simulink model "developsim"  (R2013b)
settings: Solver=ode45  StartTime=0.0  StopTime=20  RelTol=1e-3
values from neighbouring files (symbols this model uses):
  b = 0.1    [QRrunfile.m]    (also in develop.m)
  d = 0.1    [QRrunfile.m]    (also in develop.m)
  dphi0 = 0    [develop.m]
  dpsi0 = 0    [develop.m]
  dtheta0 = 0    [develop.m]
  dx0 = 0    [QRrunfile.m]    (also in develop.m)
  dy0 = 0    [QRrunfile.m]    (also in develop.m)
  dz0 = 0    [QRrunfile.m]    (also in develop.m)
  e3 = [0;0;1]    [QRrunfile.m]
  g = 9.81    [QRrunfile.m]    (also in develop.m)
  I = diag([Ixx Iyy Izz])    [QRrunfile.m]    (also in develop.m)
  Ir = 0.5    [QRrunfile.m]    (also in develop.m)
  Ixx = 0.0820    (= 0.082)    [QRrunfile.m]    (also in develop.m = 1.5)
  Iyy = 0.0845    [QRrunfile.m]    (also in develop.m = 1.5)
  Izz = .1377    (= 0.1377)    [QRrunfile.m]    (also in develop.m = 1.5)
  kOmega = kOmega_phi*eye(3)    [QRrunfile.m]
  kR = kR_phi*eye(3)    [QRrunfile.m]
  l = 0.315    [QRrunfile.m]    (also in develop.m = 0.12)
  m = 4.34    [QRrunfile.m]    (also in develop.m = 0.42)
  phi0 = 0    [develop.m]
  psi0 = 0    [develop.m]
  theta0 = 0    [develop.m]
  x0 = 0    [QRrunfile.m]    (also in develop.m)
  y0 = 0    [QRrunfile.m]    (also in develop.m)
  z0 = 0    [QRrunfile.m]    (also in develop.m)
libraries: dspsrcs4 x9, simulink x1
settings Model: Creator=Nam  LastModifiedBy=Nam
settings DebuggingCC: SolverPrmCheckMsg=none

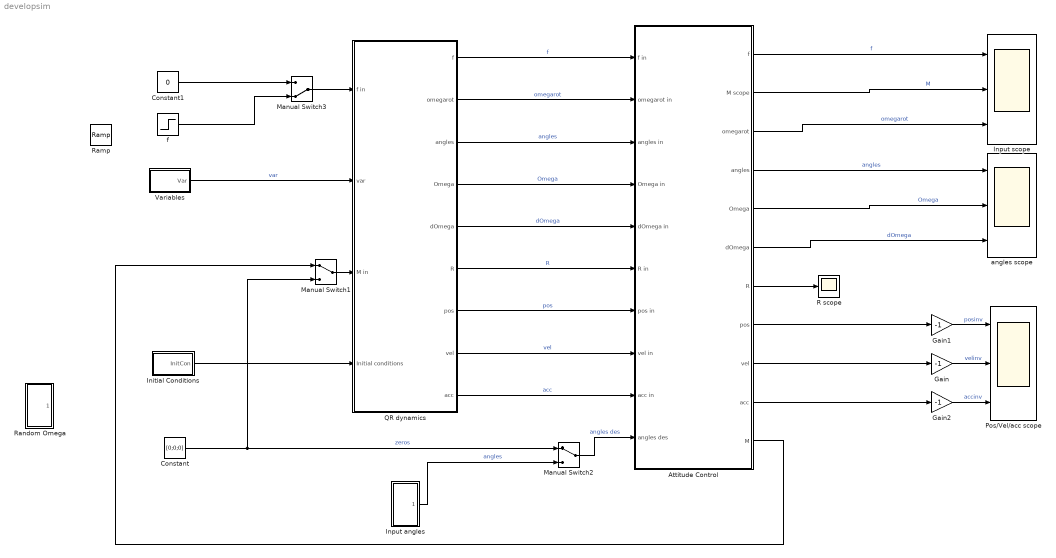
== system developsim ==
  Attitude Control : Subsystem
  Constant : Constant  Value=[0;0;0]
  Constant1 : Constant  Value=0
  Gain : Gain  Gain=-1
  Gain1 : Gain  Gain=-1
  Gain2 : Gain  Gain=-1
  Initial Conditions : Subsystem
      mask Display: disp('Initial\nConditions')
  Input angles : Subsystem
  Input scope : Scope  NumInputPorts=3
      settings: ShowLegends=on  YMin=3.91419~-1.75e+07~0  YMax=4.32621~2.5e+06~27500  SaveName=Scopeinputs
  Manual Switch1 : ManualSwitch
  Manual Switch2 : ManualSwitch
  Manual Switch3 : ManualSwitch  CurrentSetting=0
  Pos/Vel/acc scope : Scope  NumInputPorts=3
      settings: ShowLegends=on  YMin=-5~-5~-5  YMax=5~5~5  SaveName=Scopepos  SampleInput=on
  QR dynamics : Subsystem
  R scope : Scope
      settings: ShowLegends=on
  Ramp : simulink/Sources/Ramp  slope=.05  start=0  X0=m*g
  Random Omega : Subsystem
  Variables : Subsystem
      mask Display: disp('Variables')
  angles scope : Scope  NumInputPorts=3
      settings: ShowLegends=on  YMin=-5~-5~-5  YMax=5~5~5  SaveName=Scopeangles
  f : Step  Time=0  After=m*g  SampleTime=0
  wires:
  f/1 -> Manual Switch3/2
  Variables/1(Var) -> QR dynamics/2(var)  "var"
  Constant/1 -> Manual Switch2/1, Manual Switch1/2  "zeros"
  Initial Conditions/1(InitCon) -> QR dynamics/4(Initial conditions)
  QR dynamics/1(f) -> Attitude Control/1(f in)  "f"
  QR dynamics/2(omegarot) -> Attitude Control/2(omegarot in)  "omegarot"
  QR dynamics/3(angles) -> Attitude Control/3(angles in)  "angles"
  QR dynamics/5(dOmega) -> Attitude Control/5(dOmega in)  "dOmega"
  QR dynamics/6(R) -> Attitude Control/6(R in)  "R"
  QR dynamics/7(pos) -> Attitude Control/7(pos in)  "pos"
  QR dynamics/8(vel) -> Attitude Control/8(vel in)  "vel"
  QR dynamics/9(acc) -> Attitude Control/9(acc in)  "acc"
  Attitude Control/2(M scope) -> Input scope/2  "M"
  Attitude Control/3(omegarot) -> Input scope/3  "omegarot"
  Attitude Control/9(vel) -> Gain/1
  Attitude Control/7(R) -> R scope/1
  Attitude Control/10(acc) -> Gain2/1
  Attitude Control/8(pos) -> Gain1/1
  Attitude Control/1(f) -> Input scope/1  "f"
  Gain1/1 -> Pos/Vel/acc scope/1  "posinv"
  Gain/1 -> Pos/Vel/acc scope/2  "velinv"
  Gain2/1 -> Pos/Vel/acc scope/3  "accinv"
  Manual Switch1/1 -> QR dynamics/3(M in)
  Input angles/1(Out1) -> Manual Switch2/2  "angles"
  Manual Switch2/1 -> Attitude Control/10(angles des)  "angles des"
  Constant1/1 -> Manual Switch3/1
  Manual Switch3/1 -> QR dynamics/1(f in)
  Attitude Control/11(M) -> Manual Switch1/1
  QR dynamics/4(Omega) -> Attitude Control/4(Omega in)  "Omega"
  Attitude Control/4(angles) -> angles scope/1  "angles"
  Attitude Control/5(Omega) -> angles scope/2  "Omega"
  Attitude Control/6(dOmega) -> angles scope/3  "dOmega"

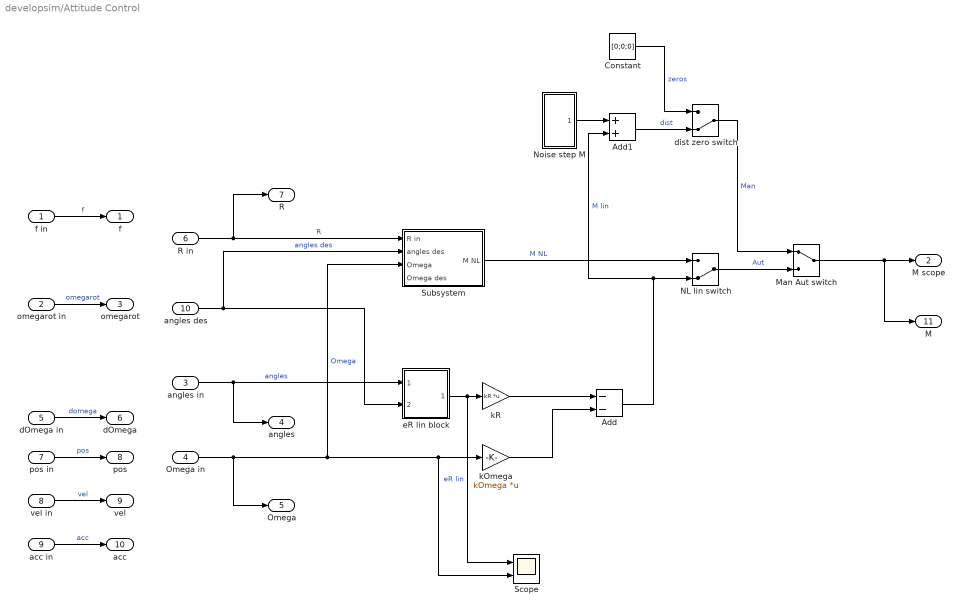
== system developsim/Attitude Control ==
  f in : Inport
  omegarot in : Inport  Port=2
  angles in : Inport  Port=3
  Omega in : Inport  Port=4
  dOmega in : Inport  Port=5
  R in : Inport  Port=6
  pos in : Inport  Port=7
  vel in : Inport  Port=8
  acc in : Inport  Port=9
  angles des : Inport  Port=10
  Add : Sum  Inputs=--
  Add1 : Sum
  Constant : Constant  Value=[0;0;0]
  Man Aut switch : ManualSwitch
  NL lin switch : ManualSwitch  CurrentSetting=0
  Noise step M : Subsystem
  Scope : Scope  NumInputPorts=2
      settings: YMin=-5~-5  YMax=5~5  SaveName=ScopeData2
  Subsystem : Subsystem
  dist zero switch : ManualSwitch  CurrentSetting=0
  eR lin block : MATLAB Function  TreatAsAtomicUnit=on
  kOmega : Gain  Gain=kOmega  Multiplication=Matrix(K*u)
  kR : Gain  Gain=kR  Multiplication=Matrix(K*u)
  f : Outport
  M scope : Outport  Port=2
  omegarot : Outport  Port=3
  angles : Outport  Port=4
  Omega : Outport  Port=5
  dOmega : Outport  Port=6
  R : Outport  Port=7
  pos : Outport  Port=8
  vel : Outport  Port=9
  acc : Outport  Port=10
  M : Outport  Port=11
  wires:
  f in/1 -> f/1  "f"
  omegarot in/1 -> omegarot/1  "omegarot"
  angles in/1 -> angles/1, eR lin block/1(angles)  "angles"
  Omega in/1 -> Subsystem/3(Omega), Scope/2, kOmega/1, Omega/1  "Omega"
  dOmega in/1 -> dOmega/1  "domega"
  pos in/1 -> pos/1  "pos"
  vel in/1 -> vel/1  "vel"
  acc in/1 -> acc/1  "acc"
  angles des/1 -> Subsystem/2(angles des), eR lin block/2(anglesdes)  "angles des"
  eR lin block/1(eRlin) -> Scope/1, kR/1  "eR lin"
  kR/1 -> Add/1
  kOmega/1 -> Add/2
  Add/1 -> NL lin switch/2, Add1/2  "M lin"
  Subsystem/1(M NL) -> NL lin switch/1  "M NL"
  R in/1 -> Subsystem/1(R in), R/1  "R"
  Noise step M/1(Out1) -> Add1/1
  NL lin switch/1 -> Man Aut switch/2  "Aut"
  Man Aut switch/1 -> M/1, M scope/1
  Constant/1 -> dist zero switch/1  "zeros"
  Add1/1 -> dist zero switch/2  "dist"
  dist zero switch/1 -> Man Aut switch/1  "Man"

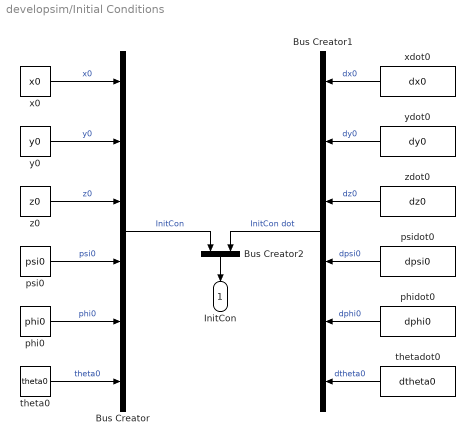
== system developsim/Initial Conditions ==
  Bus Creator : BusCreator  Inputs=6
  Bus Creator1 : BusCreator  Inputs=6
  Bus Creator2 : BusCreator  Inputs=2
  phi0 : Constant  Value=phi0
  phidot0 : Constant  Value=dphi0
  psi0 : Constant  Value=psi0
  psidot0 : Constant  Value=dpsi0
  theta0 : Constant  Value=theta0
  thetadot0 : Constant  Value=dtheta0
  x0 : Constant  Value=x0
  xdot0 : Constant  Value=dx0
  y0 : Constant  Value=y0
  ydot0 : Constant  Value=dy0
  z0 : Constant  Value=z0
  zdot0 : Constant  Value=dz0
  InitCon : Outport
  wires:
  phi0/1 -> Bus Creator/5  "phi0"
  y0/1 -> Bus Creator/2  "y0"
  psi0/1 -> Bus Creator/4  "psi0"
  x0/1 -> Bus Creator/1  "x0"
  z0/1 -> Bus Creator/3  "z0"
  theta0/1 -> Bus Creator/6  "theta0"
  Bus Creator1/1 -> Bus Creator2/2  "InitCon dot"
  psidot0/1 -> Bus Creator1/4  "dpsi0"
  xdot0/1 -> Bus Creator1/1  "dx0"
  zdot0/1 -> Bus Creator1/3  "dz0"
  ydot0/1 -> Bus Creator1/2  "dy0"
  phidot0/1 -> Bus Creator1/5  "dphi0"
  thetadot0/1 -> Bus Creator1/6  "dtheta0"
  Bus Creator2/1 -> InitCon/1
  Bus Creator/1 -> Bus Creator2/1  "InitCon"

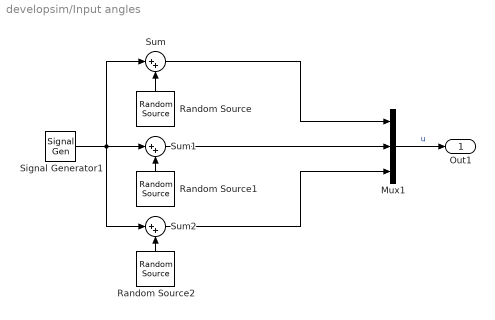
== system developsim/Input angles ==
  Mux1 : Mux  Inputs=3
  Random Source : dspsrcs4/Random Source  SrcType=Uniform  NormMethod=Ziggurat  CltLength=12  MinVal=0  MaxVal=.1  MeanVal=0  VarVal=1  RepMode=Not repeatable  rawSeed=1  IsInherit=off  SampMode=Continuous  SampTime=1  SampFrame=1  DataType=Double  OutComplex=Real
  Random Source1 : dspsrcs4/Random Source  SrcType=Uniform  NormMethod=Ziggurat  CltLength=12  MinVal=0  MaxVal=.1  MeanVal=0  VarVal=1  RepMode=Not repeatable  rawSeed=1  IsInherit=off  SampMode=Continuous  SampTime=1  SampFrame=1  DataType=Double  OutComplex=Real
  Random Source2 : dspsrcs4/Random Source  SrcType=Uniform  NormMethod=Ziggurat  CltLength=12  MinVal=0  MaxVal=.1  MeanVal=0  VarVal=1  RepMode=Not repeatable  rawSeed=1  IsInherit=off  SampMode=Continuous  SampTime=1  SampFrame=1  DataType=Double  OutComplex=Real
  Signal Generator1 : SignalGenerator  Amplitude=0.05  Frequency=50
  Sum : Sum  Inputs=|++
  Sum1 : Sum  Inputs=|++
  Sum2 : Sum  Inputs=|++
  Out1 : Outport
  wires:
  Sum/1 -> Mux1/1
  Sum2/1 -> Mux1/3
  Sum1/1 -> Mux1/2
  Random Source1/1 -> Sum1/2
  Mux1/1 -> Out1/1  "u"
  Random Source/1 -> Sum/2
  Random Source2/1 -> Sum2/2
  Signal Generator1/1 -> Sum2/1, Sum1/1, Sum/1

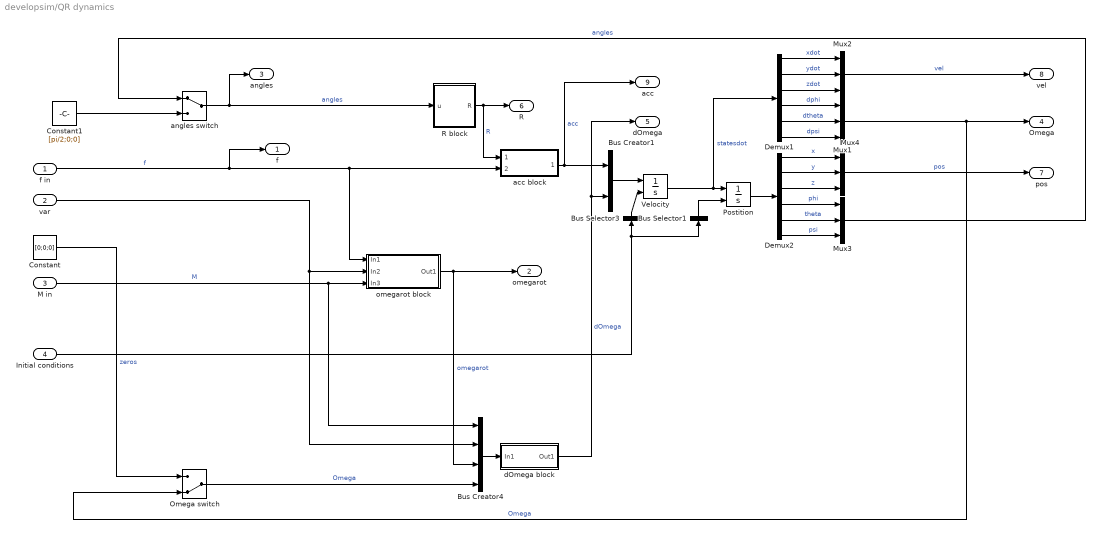
== system developsim/QR dynamics ==
  f in : Inport
  var : Inport  Port=2
  M in : Inport  Port=3
  Initial conditions : Inport  Port=4
  Bus Creator1 : BusCreator  Inputs=2
  Bus Creator4 : BusCreator
  Bus Selector1 : BusSelector  OutputSignals=InitCon.x0,InitCon.y0,InitCon.z0,InitCon.phi0,InitCon.theta0,InitCon.psi0  OutputAsBus=on
  Bus Selector3 : BusSelector  OutputSignals=InitCon dot.dx0,InitCon dot.dy0,InitCon dot.dz0,InitCon dot.dphi0,InitCon dot.dtheta0,InitCon dot.dpsi0  OutputAsBus=on
  Constant : Constant  Value=[0;0;0]
  Constant1 : Constant  Value=[pi/2;0;0]
  Demux1 : Demux  Outputs=6
  Demux2 : Demux  Outputs=6
  Mux{1..4} (4 alike) : Mux  Inputs=3
  Omega switch : ManualSwitch  CurrentSetting=0
  Postition : Integrator  InitialConditionSource=external
  R block : MATLAB Function  TreatAsAtomicUnit=on
  Velocity : Integrator  InitialConditionSource=external
  acc block : Subsystem
      mask Display: disp('[x{"}; y{"}; z{"}]','texmode','on')
  angles switch : ManualSwitch
  dOmega block : Subsystem
      mask Display: disp('[\psi{"}; \phi{"}; \theta{"}]','texmode','on')
  omegarot block : Subsystem
      mask Display: disp('[\omega_1 ; \omega_2 ; \omega_3 ; \omega_4]','texmode','on')
  f : Outport
  omegarot : Outport  Port=2
  angles : Outport  Port=3
  Omega : Outport  Port=4
  dOmega : Outport  Port=5
  R : Outport  Port=6
  pos : Outport  Port=7
  vel : Outport  Port=8
  acc : Outport  Port=9
  wires:
  Bus Selector1/1 -> Postition/2
  M in/1 -> Bus Creator4/1, omegarot block/3(In3)  "M"
  angles switch/1 -> angles/1, R block/1(u)  "angles"
  Bus Selector3/1 -> Velocity/2
  var/1 -> Bus Creator4/2, omegarot block/2(In2)
  R block/1(R) -> R/1, acc block/1(R,f,m,g1)  "R"
  Initial conditions/1 -> Bus Selector3/1, Bus Selector1/1
  acc block/1(rddotOutput) -> acc/1, Bus Creator1/1  "acc"
  Constant/1 -> Omega switch/1  "zeros"
  omegarot block/1(Out1) -> Bus Creator4/3, omegarot/1  "omegarot"
  Omega switch/1 -> Bus Creator4/4  "Omega"
  Bus Creator4/1 -> dOmega block/1(In1)
  dOmega block/1(Out1) -> dOmega/1, Bus Creator1/2  "dOmega"
  Bus Creator1/1 -> Velocity/1
  Velocity/1 -> Demux1/1, Postition/1  "statesdot"
  Demux1/4 -> Mux1/1  "dphi"
  Demux1/5 -> Mux1/2  "dtheta"
  Demux1/6 -> Mux1/3  "dpsi"
  Demux1/2 -> Mux2/2  "ydot"
  Demux1/1 -> Mux2/1  "xdot"
  Demux1/3 -> Mux2/3  "zdot"
  Demux2/4 -> Mux3/1  "phi"
  Demux2/5 -> Mux3/2  "theta"
  Demux2/6 -> Mux3/3  "psi"
  Demux2/2 -> Mux4/2  "y"
  Demux2/1 -> Mux4/1  "x"
  Demux2/3 -> Mux4/3  "z"
  Postition/1 -> Demux2/1
  Mux4/1 -> pos/1  "pos"
  Mux2/1 -> vel/1  "vel"
  Mux1/1 -> Omega switch/2, Omega/1  "Omega"
  Mux3/1 -> angles switch/1  "angles"
  f in/1 -> f/1, acc block/2(R,f,m,g), omegarot block/1(In1)  "f"
  Constant1/1 -> angles switch/2

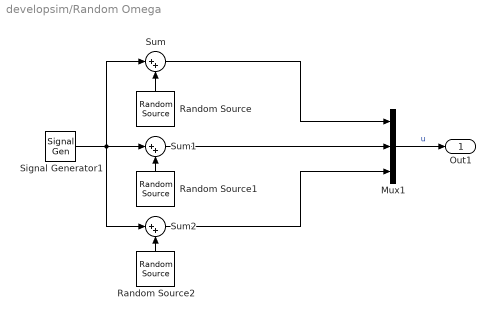
== system developsim/Random Omega ==
  Mux1 : Mux  Inputs=3
  Random Source : dspsrcs4/Random Source  SrcType=Uniform  NormMethod=Ziggurat  CltLength=12  MinVal=0  MaxVal=.1  MeanVal=0  VarVal=1  RepMode=Not repeatable  rawSeed=1  IsInherit=off  SampMode=Continuous  SampTime=1  SampFrame=1  DataType=Double  OutComplex=Real
  Random Source1 : dspsrcs4/Random Source  SrcType=Uniform  NormMethod=Ziggurat  CltLength=12  MinVal=0  MaxVal=.1  MeanVal=0  VarVal=1  RepMode=Not repeatable  rawSeed=1  IsInherit=off  SampMode=Continuous  SampTime=1  SampFrame=1  DataType=Double  OutComplex=Real
  Random Source2 : dspsrcs4/Random Source  SrcType=Uniform  NormMethod=Ziggurat  CltLength=12  MinVal=0  MaxVal=.1  MeanVal=0  VarVal=1  RepMode=Not repeatable  rawSeed=1  IsInherit=off  SampMode=Continuous  SampTime=1  SampFrame=1  DataType=Double  OutComplex=Real
  Signal Generator1 : SignalGenerator  Amplitude=0.05  Frequency=50
  Sum : Sum  Inputs=|++
  Sum1 : Sum  Inputs=|++
  Sum2 : Sum  Inputs=|++
  Out1 : Outport
  wires:
  Sum/1 -> Mux1/1
  Sum2/1 -> Mux1/3
  Sum1/1 -> Mux1/2
  Random Source1/1 -> Sum1/2
  Mux1/1 -> Out1/1  "u"
  Random Source/1 -> Sum/2
  Random Source2/1 -> Sum2/2
  Signal Generator1/1 -> Sum2/1, Sum1/1, Sum/1

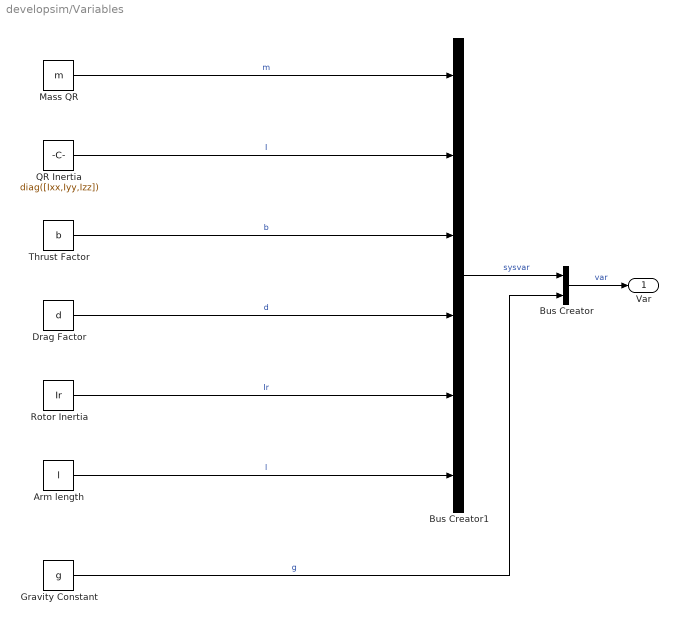
== system developsim/Variables ==
  Arm length : Constant  Value=l
  Bus Creator : BusCreator  Inputs=2
  Bus Creator1 : BusCreator  Inputs=6
  Drag Factor : Constant  Value=d
  Gravity Constant : Constant  Value=g
  Mass QR : Constant  Value=m
  QR Inertia : Constant  Value=diag([Ixx,Iyy,Izz])
  Rotor Inertia : Constant  Value=Ir
  Thrust Factor : Constant  Value=b
  Var : Outport
  wires:
  Gravity Constant/1 -> Bus Creator/2  "g"
  Bus Creator/1 -> Var/1  "var"
  Mass QR/1 -> Bus Creator1/1  "m"
  Arm length/1 -> Bus Creator1/6  "l"
  Rotor Inertia/1 -> Bus Creator1/5  "Ir"
  QR Inertia/1 -> Bus Creator1/2  "I"
  Bus Creator1/1 -> Bus Creator/1  "sysvar"
  Thrust Factor/1 -> Bus Creator1/3  "b"
  Drag Factor/1 -> Bus Creator1/4  "d"

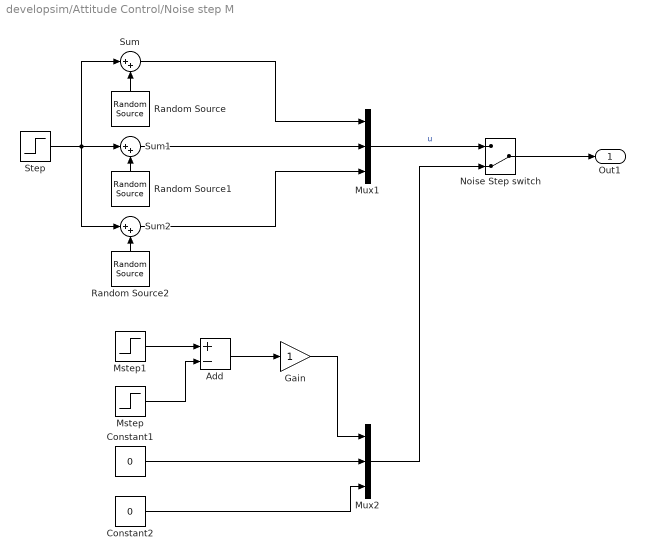
== system developsim/Attitude Control/Noise step M ==
  Add : Sum  Inputs=+-
  Constant1 : Constant  Value=0
  Constant2 : Constant  Value=0
  Gain : Gain
  Mstep : Step  Time=6  SampleTime=0
  Mstep1 : Step  Time=5  SampleTime=0
  Mux1 : Mux  Inputs=3
  Mux2 : Mux  Inputs=3
  Noise Step switch : ManualSwitch  CurrentSetting=0
  Random Source : dspsrcs4/Random Source  SrcType=Uniform  NormMethod=Ziggurat  CltLength=12  MinVal=0  MaxVal=.1  MeanVal=0  VarVal=1  RepMode=Not repeatable  rawSeed=1  IsInherit=off  SampMode=Continuous  SampTime=1  SampFrame=1  DataType=Double  OutComplex=Real
  Random Source1 : dspsrcs4/Random Source  SrcType=Uniform  NormMethod=Ziggurat  CltLength=12  MinVal=0  MaxVal=.1  MeanVal=0  VarVal=1  RepMode=Not repeatable  rawSeed=1  IsInherit=off  SampMode=Continuous  SampTime=1  SampFrame=1  DataType=Double  OutComplex=Real
  Random Source2 : dspsrcs4/Random Source  SrcType=Uniform  NormMethod=Ziggurat  CltLength=12  MinVal=0  MaxVal=.1  MeanVal=0  VarVal=1  RepMode=Not repeatable  rawSeed=1  IsInherit=off  SampMode=Continuous  SampTime=1  SampFrame=1  DataType=Double  OutComplex=Real
  Step : Step  Time=0  After=0  SampleTime=0
  Sum : Sum  Inputs=|++
  Sum1 : Sum  Inputs=|++
  Sum2 : Sum  Inputs=|++
  Out1 : Outport
  wires:
  Sum/1 -> Mux1/1
  Sum2/1 -> Mux1/3
  Sum1/1 -> Mux1/2
  Random Source1/1 -> Sum1/2
  Mux1/1 -> Noise Step switch/1  "u"
  Random Source/1 -> Sum/2
  Random Source2/1 -> Sum2/2
  Step/1 -> Sum2/1, Sum1/1, Sum/1
  Constant1/1 -> Mux2/2
  Constant2/1 -> Mux2/3
  Mux2/1 -> Noise Step switch/2
  Noise Step switch/1 -> Out1/1
  Mstep1/1 -> Add/1
  Mstep/1 -> Add/2
  Add/1 -> Gain/1
  Gain/1 -> Mux2/1

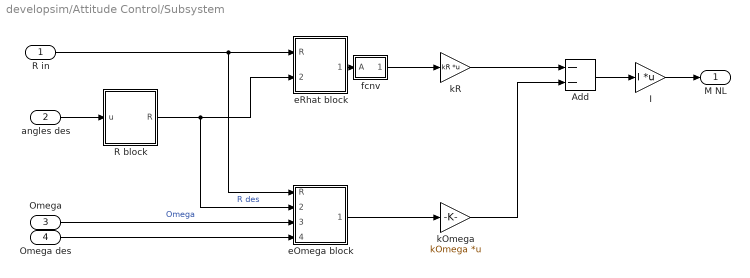
== system developsim/Attitude Control/Subsystem ==
  R in : Inport
  angles des : Inport  Port=2
  Omega : Inport  Port=3
  Omega des : Inport  Port=4
  Add : Sum  Inputs=--
  I : Gain  Gain=I  Multiplication=Matrix(K*u)
  R block : MATLAB Function  TreatAsAtomicUnit=on
  eOmega block : MATLAB Function  TreatAsAtomicUnit=on
  eRhat block : MATLAB Function  TreatAsAtomicUnit=on
  fcnv : MATLAB Function  TreatAsAtomicUnit=on
  kOmega : Gain  Gain=kOmega  Multiplication=Matrix(K*u)
  kR : Gain  Gain=kR  Multiplication=Matrix(K*u)
  M NL : Outport
  wires:
  R in/1 -> eOmega block/1(R), eRhat block/1(R)
  R block/1(R) -> eOmega block/2(Rdes), eRhat block/2(Rdes)  "R des"
  eRhat block/1(eRhat) -> fcnv/1(A)
  angles des/1 -> R block/1(u)
  fcnv/1(fcnv) -> kR/1
  kR/1 -> Add/1
  kOmega/1 -> Add/2
  Omega/1 -> eOmega block/3(Omega)  "Omega"
  Omega des/1 -> eOmega block/4(Omegades)
  eOmega block/1(eOmega) -> kOmega/1
  Add/1 -> I/1
  I/1 -> M NL/1

== system developsim/QR dynamics/acc block ==
  R,f,m,g1 : Inport
  R,f,m,g : Inport  Port=2
  Constant : Constant  Value=m
  Constant1 : Constant  Value=g
  fcnddr : MATLAB Function  TreatAsAtomicUnit=on
  rddotOutput : Outport
  wires:
  fcnddr/1(ddr) -> rddotOutput/1  "ddr"
  R,f,m,g/1 -> fcnddr/2(f)  "f"
  R,f,m,g1/1 -> fcnddr/1(R)  "R"
  Constant/1 -> fcnddr/3(m)
  Constant1/1 -> fcnddr/4(g)

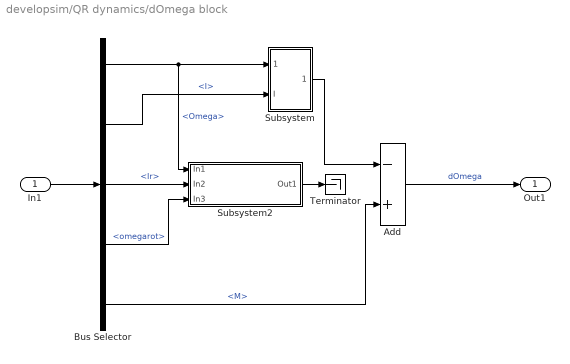
== system developsim/QR dynamics/dOmega block ==
  In1 : Inport
  Add : Sum  Inputs=-+
  Bus Selector : BusSelector  OutputSignals=Omega,var.sysvar.I,var.sysvar.Ir,omegarot,M
  Subsystem : Subsystem
      mask Display: disp('\Omega \times I\Omega','texmode','on')
  Subsystem2 : Subsystem
      mask Display: disp('\tau_G=\Sigma I_R(\omega \times e_3) \omega_i ','texmode','on')
  Terminator : Terminator
  Out1 : Outport
  wires:
  In1/1 -> Bus Selector/1
  Add/1 -> Out1/1  "dOmega"
  Bus Selector/1 -> Subsystem/1(Omega), Subsystem2/1(In1)  "<Omega>"
  Bus Selector/2 -> Subsystem/2(I)  "<I>"
  Subsystem/1(Out1) -> Add/1
  Bus Selector/3 -> Subsystem2/2(In2)  "<Ir>"
  Bus Selector/4 -> Subsystem2/3(In3)  "<omegarot>"
  Bus Selector/5 -> Add/2  "<M>"
  Subsystem2/1(Out1) -> Terminator/1

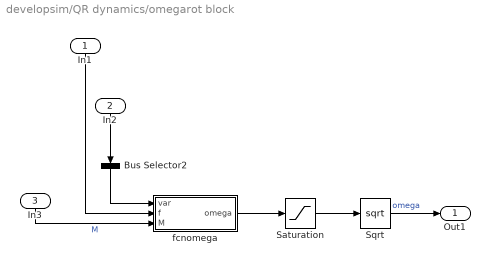
== system developsim/QR dynamics/omegarot block ==
  In1 : Inport
  In2 : Inport  Port=2
  In3 : Inport  Port=3
  Bus Selector2 : BusSelector  OutputSignals=sysvar.b,sysvar.d,sysvar.l  OutputAsBus=on
  Saturation : Saturate  UpperLimit=inf  LowerLimit=0
  Sqrt : Sqrt  SaturateOnIntegerOverflow=on
  fcnomega : MATLAB Function  TreatAsAtomicUnit=on
  Out1 : Outport
  wires:
  In3/1 -> fcnomega/3(M)  "M"
  In1/1 -> fcnomega/2(f)
  In2/1 -> Bus Selector2/1
  Bus Selector2/1 -> fcnomega/1(var)
  Sqrt/1 -> Out1/1  "omega"
  fcnomega/1(omega) -> Saturation/1
  Saturation/1 -> Sqrt/1

== system developsim/QR dynamics/dOmega block/Subsystem ==
  Omega : Inport
  I : Inport  Port=2
  Product : Product  Inputs=3  Multiplication=Matrix(*)
  fcnhat : MATLAB Function  TreatAsAtomicUnit=on
  Out1 : Outport
  wires:
  Omega/1 -> Product/3, fcnhat/1(A)
  fcnhat/1(fcnhat) -> Product/1
  I/1 -> Product/2
  Product/1 -> Out1/1

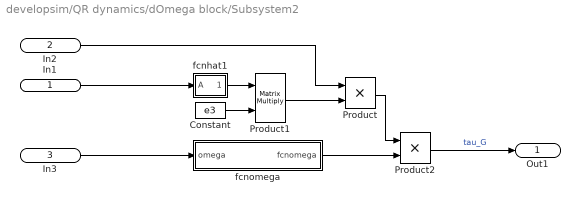
== system developsim/QR dynamics/dOmega block/Subsystem2 ==
  In1 : Inport
  In2 : Inport  Port=2
  In3 : Inport  Port=3
  Constant : Constant  Value=e3
  Product : Product
  Product1 : Product  Multiplication=Matrix(*)
  Product2 : Product
  fcnhat1 : MATLAB Function  TreatAsAtomicUnit=on
  fcnomega : MATLAB Function  TreatAsAtomicUnit=on
  Out1 : Outport
  wires:
  Product2/1 -> Out1/1  "tau_G"
  In2/1 -> Product/1
  fcnomega/1(fcnomega) -> Product2/2
  Product1/1 -> Product/2
  In3/1 -> fcnomega/1(omega)
  In1/1 -> fcnhat1/1(A)
  fcnhat1/1(fcnhat) -> Product1/1
  Constant/1 -> Product1/2
  Product/1 -> Product2/1

== matlab function developsim/QR dynamics/omegarot block/fcnomega ==
  data: var input; f input; M input size=[3 1]; omega output
function omega = fcn(var,f,M)
%omega = [omega_1^2;omega_2^2;omega_3^2;omega_4^2]

b = var(1);
d = var(2);
l = var(3);

%check if Gamma is invertible?
Gamma = [b b b b;0 -l*b 0 l*b;l*b 0 -l*b 0;-d d -d d];

QRinput = [f;M];

omega = Gamma\QRinput;

== matlab function developsim/QR dynamics/acc block/fcnddr ==
  data: R input size=[3 3]; ddr output size=[3 1]; f input size=1; m input; g input
function ddr = fcn(R,f,m,g)
%ddr = [xddot; yddot; zddot]
%e3 downwards
%m*vdot = g*e_3-f/m*R*e3



ddr = ([0;0;m*g]-f*R*[0;0;1]) / m;

== matlab function developsim/QR dynamics/R block ==
  data: u input; R output
function R = fcnR(u)
% Z-X-Y psi-phi-theta
% u1 = phi, 
% u2 = theta, 
% u3 = psi

phi        = u(1);
theta      = u(2);
psi        = u(3);

R          = [cos(psi)*cos(theta)-sin(phi)*sin(psi)*sin(theta)   -cos(phi)*sin(psi)   cos(psi)*sin(theta)+cos(theta)*sin(phi)*sin(psi);
              cos(theta)*sin(psi)+cos(psi)*sin(phi)*sin(theta)    cos(phi)*cos(psi)   sin(psi)*sin(theta)-cos(psi)*cos(theta)*sin(phi);
             -cos(phi)*sin(theta)                                 sin(phi)            cos(phi)*cos(theta)];

== matlab function developsim/QR dynamics/dOmega block/Subsystem2/fcnhat1 ==
  data: A input; fcnhat output
function fcnhat = fcn(A)

a = A(1);
b = A(2);
c = A(3);
fcnhat = [0 -c b; 
          c 0 -a;
         -b a 0];

== matlab function developsim/Attitude Control/Subsystem/R block ==
  data: u input; R output
function R = fcnR(u)
% Z-X-Y psi-phi-theta
% u1 = phi, 
% u2 = theta, 
% u3 = psi

phi        = u(1);
theta      = u(2);
psi        = u(3);

R          = [cos(psi)*cos(theta)-sin(phi)*sin(psi)*sin(theta)   -cos(phi)*sin(psi)   cos(psi)*sin(theta)+cos(theta)*sin(phi)*sin(psi);
              cos(theta)*sin(psi)+cos(psi)*sin(phi)*sin(theta)    cos(phi)*cos(psi)   sin(psi)*sin(theta)-cos(psi)*cos(theta)*sin(phi);
             -cos(phi)*sin(theta)                                 sin(phi)            cos(phi)*cos(theta)];

== matlab function developsim/QR dynamics/dOmega block/Subsystem2/fcnomega ==
  data: omega input; fcnomega output
function fcnomega = fcn(omega)

fcnomega = omega(2)+omega(4)-omega(1)-omega(3);

== matlab function developsim/QR dynamics/dOmega block/Subsystem/fcnhat ==
  data: A input; fcnhat output
function fcnhat = fcn(A)

a = A(1);
b = A(2);
c = A(3);
fcnhat = [0 -c b; 
          c 0 -a;
         -b a 0];

== matlab function developsim/Attitude Control/Subsystem/eRhat block ==
  data: R input size=[3 3]; Rdes input size=[3 3]; eRhat output size=[3 3]
function eRhat = fcnR(R,Rdes)
% Z-X-Y psi-phi-theta

eRhat = 0.5*(Rdes'*R-R'*Rdes);

== matlab function developsim/Attitude Control/Subsystem/fcnv ==
  data: A input size=[3 3]; fcnv output size=[3 1]
function fcnv = fcn(A)
% Inverse hat function

a    = A(6);
b    = -A(3);
c    = A(2);

fcnv = [a;b;c];

== matlab function developsim/Attitude Control/eR lin block ==
  data: angles input size=[3 1]; anglesdes input size=[3 1]; eRlin output size=[3 1]
function eRlin = fcnR(angles,anglesdes)
% Z-X-Y psi-phi-theta
% Rdes =  R(psi0+dpsi, dphi, dtheta)
% R = R(psi0,0,0)

dphi   = anglesdes(1) - angles(1);
dtheta = anglesdes(2) - angles(2);
dpsi   = anglesdes(3) - angles(3);

% eRlin  = [dphi; dtheta; dpsi];
% Of toch: 
eRlin  = [-dphi; -dtheta; -dpsi];

== matlab function developsim/Attitude Control/Subsystem/eOmega block ==
  data: R input size=[3 3]; Rdes input size=[3 3]; eOmega output size=[3 1]; Omega input size=[3 1]; Omegades input size=[3 1]
function eOmega = fcnR(R,Rdes,Omega,Omegades)
% Z-X-Y psi-phi-theta

eOmega = Omega - R'*Rdes*Omegades;
